simulink library "Qconj"  (R2015b)
settings: Solver=VariableStepAuto  StartTime=0.0  StopTime=10.0  RelTol=1e-3
settings Model: Creator=y.akisheva  LastModifiedBy=y.akisheva

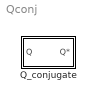
== system Qconj ==
  Q_conjugate : Subsystem

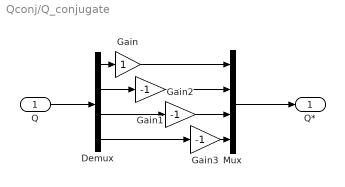
== system Qconj/Q_conjugate ==
  Q : Inport
  Demux : Demux
  Gain : Gain
  Gain1 : Gain  Gain=-1
  Gain2 : Gain  Gain=-1
  Gain3 : Gain  Gain=-1
  Mux : Mux
  Q* : Outport
  wires:
  Gain3/1 -> Mux/4
  Q/1 -> Demux/1
  Gain2/1 -> Mux/3
  Demux/2 -> Gain1/1
  Demux/3 -> Gain2/1
  Gain1/1 -> Mux/2
  Demux/4 -> Gain3/1
  Mux/1 -> Q*/1
  Gain/1 -> Mux/1
  Demux/1 -> Gain/1
